simulink model "Problem_8"  (R2020a)
settings: Solver=VariableStepAuto  StartTime=0.0  StopTime=10.0  RelTol=1e-3
settings Model: Creator=user  LastModifiedBy=user

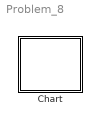
== system Problem_8 ==
  Chart : Stateflow chart  TreatAsAtomicUnit=on

== stateflow chart Problem_8/Chart ==
  state Active
    state GroundFloor
    state FirstFloor
    state SecondFloor
    state FifthFloor
    state FourthFloor
    state ThirdFloor
    (default) -> GroundFloor
    FirstFloor -> SecondFloor [order 2]
    GroundFloor -> FirstFloor : [button == 1]
    SecondFloor -> FirstFloor [order 1]
    FirstFloor -> GroundFloor [order 1] : [button == 0]
    ThirdFloor -> SecondFloor [order 1]
    SecondFloor -> ThirdFloor [order 2]
    ThirdFloor -> FourthFloor [order 2]
    FourthFloor -> FifthFloor [order 2]
    FifthFloor -> FourthFloor
    FourthFloor -> ThirdFloor [order 1]
  state ForceStop
  (default) -> Active
  Active -> ForceStop : [error == 1]
  ForceStop -> Active : [error == 0]
